simulink model "RL4RboticFirstExercise"  (R2017b)
settings: Solver=VariableStepAuto  StartTime=0.0  StopTime=20  RelTol=1e-3
undefined symbols (not defined in the file or in its folder): L
settings Model: Creator=shangyingao  LastModifiedBy=shangyingao

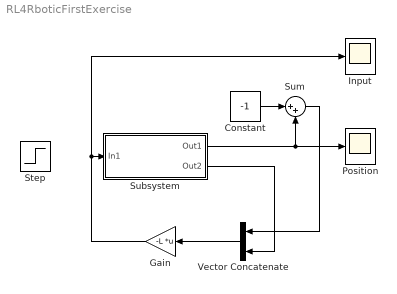
== system RL4RboticFirstExercise ==
  Constant : Constant  Value=-1
  Gain : Gain  Gain=-L  Multiplication=Matrix(K*u)
  "Input " : Scope
  Position : Scope
  Step : Step  SampleTime=0
  Subsystem : Subsystem
  Sum : Sum  Inputs=|++
  Vector Concatenate : Concatenate
  wires:
  Subsystem/2(Out2) -> Vector Concatenate/2
  Vector Concatenate/1 -> Gain/1
  Gain/1 -> "Input "/1, Subsystem/1(In1)
  Constant/1 -> Sum/1
  Subsystem/1(Out1) -> Position/1, Sum/2
  Sum/1 -> Vector Concatenate/1

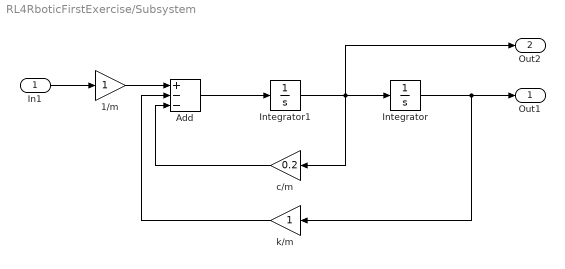
== system RL4RboticFirstExercise/Subsystem ==
  In1 : Inport
  1/m : Gain
  Add : Sum  Inputs=+--
  Integrator : Integrator
  Integrator1 : Integrator
  c/m : Gain  Gain=0.2
  k/m : Gain
  Out1 : Outport
  Out2 : Outport  Port=2
  wires:
  Integrator1/1 -> c/m/1, Out2/1, Integrator/1
  c/m/1 -> Add/3
  Integrator/1 -> k/m/1, Out1/1
  k/m/1 -> Add/2
  Add/1 -> Integrator1/1
  1/m/1 -> Add/1
  In1/1 -> 1/m/1
